simulink model "model_2"  (R2021a)
settings: Solver=FixedStepAuto  StartTime=0.0  StopTime=2  FixedStep=step  RelTol=1e-3
values from neighbouring files (symbols this model uses):
  qc = robot.ikine(Tcart,q0,'mask',mask)    [TP.m]
undefined symbols (not defined in the file or in its folder): Kp, Kv
libraries: roblocks x5, simulink x1
settings Model: Creator=ohvic  LastModifiedBy=ohvic

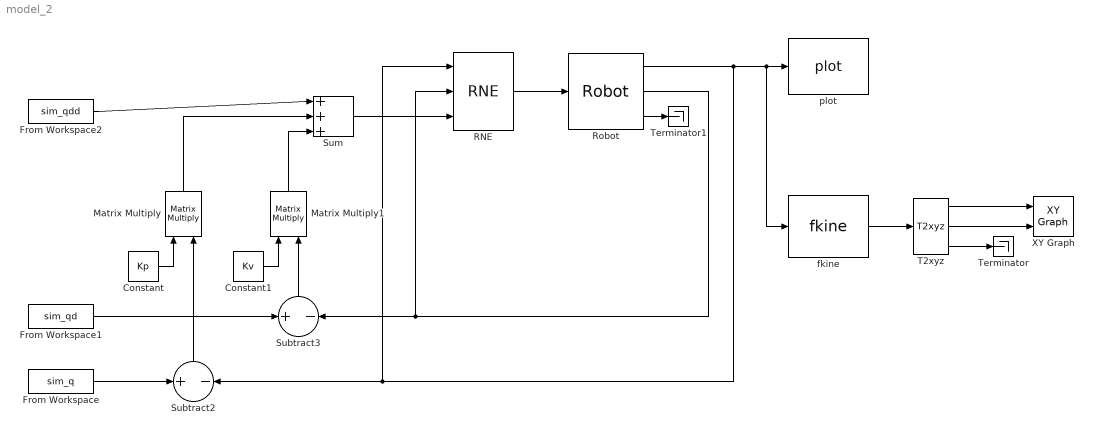
== system model_2 ==
  Constant : Constant  Value=Kp
  Constant1 : Constant  Value=Kv
  From Workspace : FromWorkspace  VariableName=sim_q  SampleTime=step
  From Workspace1 : FromWorkspace  VariableName=sim_qd  SampleTime=step
  From Workspace2 : FromWorkspace  VariableName=sim_qdd  SampleTime=step
  Matrix Multiply : Product  Multiplication=Matrix(*)
  Matrix Multiply1 : Product  Multiplication=Matrix(*)
  RNE : roblocks/Arm/RNE  robot=robot  grav=[0 0 9.81]
  Robot : roblocks/Arm/Robot  robot=robot  q0=qc(1,:)
  Subtract2 : Sum  Inputs=+-
  Subtract3 : Sum  Inputs=+-
  Sum : Sum  Inputs=|+++
  T2xyz : roblocks/Toolbox/T2xyz
  Terminator : Terminator
  Terminator1 : Terminator
  XY Graph : simulink/Sinks/XY Graph  xmin=-2  xmax=2  ymin=-2  ymax=2  st=-1
  fkine : roblocks/Arm/fkine  robot=robot
  plot : roblocks/Arm/plot  robot=robot  fps=25  holdplot=off
  wires:
  Constant/1 -> Matrix Multiply/1
  Constant1/1 -> Matrix Multiply1/1
  From Workspace/1 -> Subtract2/1
  From Workspace1/1 -> Subtract3/1
  Subtract2/1 -> Matrix Multiply/2
  Subtract3/1 -> Matrix Multiply1/2
  From Workspace2/1 -> Sum/1
  Matrix Multiply/1 -> Sum/2
  Matrix Multiply1/1 -> Sum/3
  Robot/3 -> Terminator1/1
  T2xyz/1 -> XY Graph/1
  T2xyz/2 -> XY Graph/2
  fkine/1 -> T2xyz/1
  T2xyz/3 -> Terminator/1
  Robot/2 -> Subtract3/2, RNE/2
  Robot/1 -> fkine/1, plot/1, Subtract2/2, RNE/1
  Sum/1 -> RNE/3
  RNE/1 -> Robot/1
